simulink model "ar_lht_hw_target"  (R2018a)
settings: Solver=VariableStepAuto  StartTime=0.0  StopTime=ts*4+(526+25)*4*T  RelTol=1e-3  EnableMultiTasking=on
PreLoadFcn:
  | currentDir  = pwd;
  | filesepIdx   = strfind(currentDir, filesep);
  | newDir = currentDir(1:filesepIdx(end)-7);
  | 
  | addpath([newDir, '\scripts']);
InitFcn:
  | setup;
  | pre_processing;
values from neighbouring files (symbols this model uses):
  deltaTheta = 1    [setup.m]
  fps = f/((height)*(width))    (= 184.377034505)    [setup.m]
  height = 768    [setup.m]
  K = (maxTheta + deltaTheta)/R    (= 45)    [setup.m]
  maxRho = ceil(sqrt((height/2)^2+(width/2)^2))    [setup.m]
  maxTheta = 179    [setup.m]
  R = 4    [setup.m]
  T = 1/f    (= 6.89655172414e-09)    [setup.m]
  width = 1024    [setup.m]
libraries: xbsIndex_r4 x220, hdlsllib x6, visionhdlio x1, visionsources x1
(part 1 of 2)
settings Model: Creator=David Northcote  LastModifiedBy=rgb11127
settings OptimizationCC: LifeSpan=inf
settings DebuggingCC: SFUnexpectedBacktrackingDiag=warning  SFNoUnconditionalDefaultTransitionDiag=warning  SFExecutionAtInitializationDiag=none
settings CodeAppCC: StateflowObjectComments=on
settings GRTTargetCC: TargetLangStandard=C89/C90 (ANSI)  GeneratePreprocessorConditionals=Disable all
settings ConfigComp: CovMetricSettings=dw  CovHtmlReporting=on  CovSaveCumulativeToWorkspaceVar=on  CovSaveSingleToWorkspaceVar=on  CovExternalEMLEnable=off

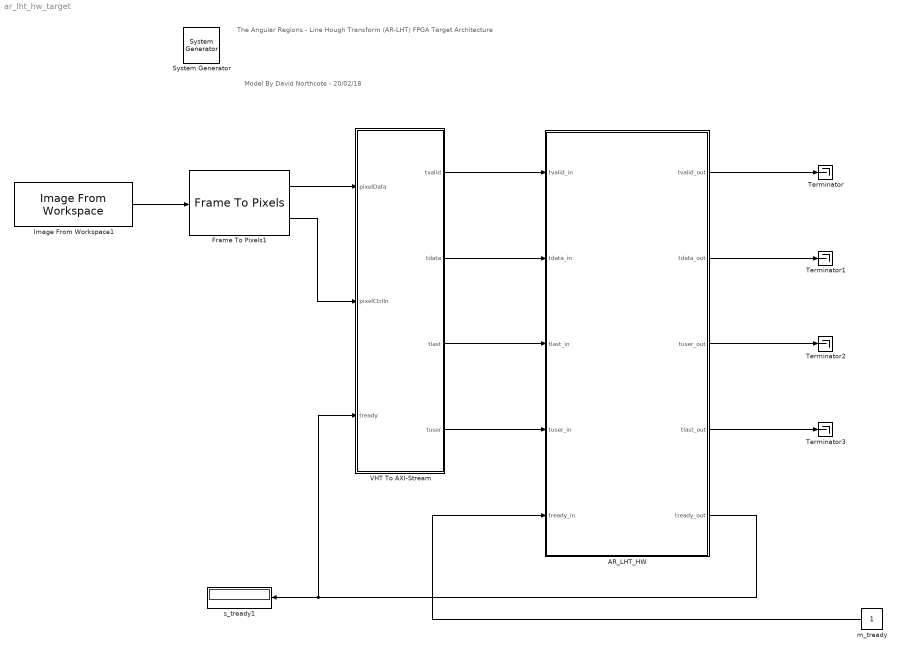
== system ar_lht_hw_target ==
  note: Model By David Northcote - 20/02/18
  note: The Angular Regions - Line Hough Transform (AR-LHT)
      | FPGA Target Architecture
  " System Generator" : xbsIndex_r4/ System Generator  Tag=genX  xilinxfamily=zynq  part=xc7z010  speed=-1  package=clg400  synthesis_tool=Vivado  clock_wrapper=Clock Enables  directory=./netlist  proj_type=Vivado  Synth_file=Vivado Synthesis Defaults  Impl_file=Vivado Implementation Defaults  testbench=off  simulink_period=T  sysclk_period=T*1e9  dcm_input_clock_period=10  incr_netlist=off  trim_vbits=Everywhere in SubSystem  dbl_ovrd=According to Block Masks  core_generation=According to Block Masks  run_coregen=off  deprecated_control=off  eval_field=0  block_type=sysgen
  AR_LHT_HW : Subsystem
  Frame To Pixels1 : visionhdlio/Frame To Pixels  NumComponents=1  VideoFormat=Custom  ActivePixelsPerLine=width  ActiveVideoLines=height  TotalPixelsPerLine=width  TotalVideoLines=height  StartingActiveLine=1  FrontPorch=0  SampleTime=0
      settings: SourceProductName=Vision HDL Toolbox  SourceProductBaseCode=VT
  Image From Workspace1 : visionsources/Image From Workspace  Tag=vipblks_nd  ImageValue=InputImage  Ts=1/fps  imagePorts=One multidimensional signal  OutPortLabels=R|G|B  ImageDataType=Inherit from 'Value'  Signed=on  WordLength=16  sdImageDataType=sfix(16)  FractionLengthMode=User-defined  FractionLength=15
      settings: SourceProductName=Computer Vision System Toolbox  SourceProductBaseCode=VP
  Terminator{,1..3} (4 alike) : Terminator
  VHT To AXI-Stream : Subsystem
  m_tready : Constant  OutDataTypeStr=boolean  SampleTime=T
  s_tready1 : Display
  wires:
  m_tready/1 -> AR_LHT_HW/5(tready_in)
  AR_LHT_HW/4(tlast_out) -> Terminator3/1
  AR_LHT_HW/3(tuser_out) -> Terminator2/1
  AR_LHT_HW/2(tdata_out) -> Terminator1/1
  AR_LHT_HW/1(tvalid_out) -> Terminator/1
  AR_LHT_HW/5(tready_out) -> s_tready1/1, VHT To AXI-Stream/3(tready)
  VHT To AXI-Stream/1(tvalid) -> AR_LHT_HW/1(tvalid_in)
  VHT To AXI-Stream/3(tlast) -> AR_LHT_HW/3(tlast_in)
  VHT To AXI-Stream/2(tdata) -> AR_LHT_HW/2(tdata_in)
  VHT To AXI-Stream/4(tuser) -> AR_LHT_HW/4(tuser_in)
  Frame To Pixels1/1 -> VHT To AXI-Stream/1(pixelData)
  Frame To Pixels1/2 -> VHT To AXI-Stream/2(pixelCtrlIn)
  Image From Workspace1/1 -> Frame To Pixels1/1

== system ar_lht_hw_target/AR_LHT_HW ==
  tvalid_in : Inport
  tdata_in : Inport  Port=2
  tlast_in : Inport  Port=3
  tuser_in : Inport  Port=4
  tready_in : Inport  Port=5
  DUT : Subsystem
  M_AXIS : Subsystem
  S_AXIS : Subsystem
  tvalid_out : Outport
  tdata_out : Outport  Port=2
  tuser_out : Outport  Port=3
  tlast_out : Outport  Port=4
  tready_out : Outport  Port=5
  wires:
  DUT/5(tready_out) -> S_AXIS/5(tready_in)
  M_AXIS/1(tready_out) -> DUT/5(tready_in)
  DUT/1(tvalid_out) -> M_AXIS/1(tvalid_in)
  DUT/2(tdata_out) -> M_AXIS/2(tdata_in)
  DUT/3(tlast_out) -> M_AXIS/3(tlast_in)
  DUT/4(tuser_out) -> M_AXIS/4(tuser_in)
  S_AXIS/2(tdata_out) -> DUT/2(tdata_in)
  S_AXIS/1(tvalid_out) -> DUT/1(tvalid_in)
  S_AXIS/3(tlast_out) -> DUT/3(tlast_in)
  S_AXIS/4(tuser_out) -> DUT/4(tuser_in)
  M_AXIS/4(tuser_out) -> tuser_out/1
  S_AXIS/5(tready_out) -> tready_out/1
  M_AXIS/5(tlast_out) -> tlast_out/1
  M_AXIS/3(tdata_out) -> tdata_out/1
  tready_in/1 -> M_AXIS/5(tready_in)
  M_AXIS/2(tvalid_out) -> tvalid_out/1
  tlast_in/1 -> S_AXIS/3(tlast_in)
  tvalid_in/1 -> S_AXIS/1(tvalid_in)
  tuser_in/1 -> S_AXIS/4(tuser_in)
  tdata_in/1 -> S_AXIS/2(tdata_in)

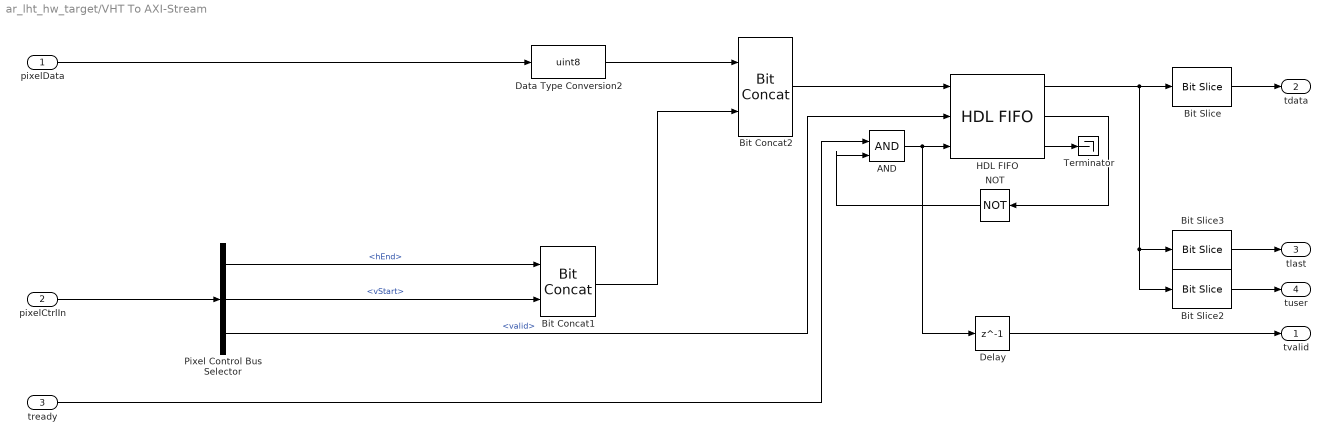
== system ar_lht_hw_target/VHT To AXI-Stream ==
  pixelData : Inport
  pixelCtrlIn : Inport  Port=2
  tready : Inport  Port=3
  AND : Logic  IconShape=distinctive  AllPortsSameDT=off  OutDataTypeStr=boolean
  Bit Concat1 : hdlsllib/Logic and Bit Operations/Bit Concat  numInputs=2
      settings: SourceProductName=HDL Coder  SourceProductBaseCode=HD
  Bit Concat2 : hdlsllib/Logic and Bit Operations/Bit Concat  numInputs=2
      settings: SourceProductName=HDL Coder  SourceProductBaseCode=HD
  Bit Slice : hdlsllib/Logic and Bit Operations/Bit Slice  lidx=9  ridx=2
  Bit Slice2 : hdlsllib/Logic and Bit Operations/Bit Slice  lidx=0  ridx=0
  Bit Slice3 : hdlsllib/Logic and Bit Operations/Bit Slice  lidx=1  ridx=1
  Data Type Conversion2 : DataTypeConversion  OutDataTypeStr=uint8
  Delay : Delay  DelayLength=1
  HDL FIFO : hdlsllib/HDL RAMs/HDL FIFO  fifo_size=1024  ratio=1  push_msg=Error  pop_msg=Error  show_empty=on  show_full=on  show_num=off
      settings: SourceProductName=HDL Coder  SourceProductBaseCode=HD
  NOT : Logic  Operator=NOT  IconShape=distinctive  AllPortsSameDT=off  OutDataTypeStr=boolean
  Pixel Control Bus Selector : BusSelector  OutputSignals=hEnd,vStart,valid
  Terminator : Terminator
  tvalid : Outport
  tdata : Outport  Port=2
  tlast : Outport  Port=3
  tuser : Outport  Port=4
  wires:
  pixelData/1 -> Data Type Conversion2/1
  pixelCtrlIn/1 -> Pixel Control Bus Selector/1
  Bit Concat2/1 -> HDL FIFO/1
  Data Type Conversion2/1 -> Bit Concat2/1
  Bit Concat1/1 -> Bit Concat2/2
  HDL FIFO/1 -> Bit Slice3/1, Bit Slice2/1, Bit Slice/1
  tready/1 -> AND/1
  HDL FIFO/2 -> NOT/1
  NOT/1 -> AND/2
  Bit Slice/1 -> tdata/1
  Bit Slice3/1 -> tlast/1
  Bit Slice2/1 -> tuser/1
  AND/1 -> Delay/1, HDL FIFO/3
  Pixel Control Bus Selector/1 -> Bit Concat1/1  "<hEnd>"
  Pixel Control Bus Selector/2 -> Bit Concat1/2  "<vStart>"
  Pixel Control Bus Selector/3 -> HDL FIFO/2  "<valid>"
  Delay/1 -> tvalid/1
  HDL FIFO/3 -> Terminator/1

== system ar_lht_hw_target/AR_LHT_HW/DUT ==
  tvalid_in : Inport
  tdata_in : Inport  Port=2
  tlast_in : Inport  Port=3
  tuser_in : Inport  Port=4
  tready_in : Inport  Port=5
  AXI FIFO : xbsIndex_r4/AXI FIFO  input_depth_axis=16  actual_fifo_depth_label=18  enable_tdata=on  enable_tdest=off  enable_tstrb=off  enable_tready=on  enable_tid=off  enable_tuser=on  enable_tkeep=off  enable_tlast=on  has_aresetn=off  enable_data_counts_axis=off  fifo_implementation_type_axis=Common Clock Distributed RAM  trim_axipin_name=on  programmable_full_type_axis=Full  full_threshold_assert_value_axis=0  programmable_empty_type_axis=Empty  empty_threshold_assert_value_axis=1022  underflow_flag_axi=0  underflow_sense_axi=Active High  overflow_flag_axi=0  overflow_sense_axi=Active High  block_type=axi_fifo
  Algorithm : Subsystem
  tvalid_out : Outport
  tdata_out : Outport  Port=2
  tlast_out : Outport  Port=3
  tuser_out : Outport  Port=4
  tready_out : Outport  Port=5
  wires:
  tvalid_in/1 -> Algorithm/2(tvalid_in)
  tready_in/1 -> Algorithm/1(tready_in)
  tlast_in/1 -> Algorithm/4(tlast_in)
  tuser_in/1 -> Algorithm/5(tuser_in)
  tdata_in/1 -> Algorithm/3(tdata_in)
  AXI FIFO/4 -> tuser_out/1
  AXI FIFO/3 -> tlast_out/1
  AXI FIFO/1 -> tvalid_out/1
  AXI FIFO/2 -> tdata_out/1
  AXI FIFO/5 -> tready_out/1
  Algorithm/5(tuser_out) -> AXI FIFO/5
  Algorithm/4(tlast_out) -> AXI FIFO/4
  Algorithm/3(tdata_out) -> AXI FIFO/3
  Algorithm/2(tvalid_out) -> AXI FIFO/2
  Algorithm/1(tready_out) -> AXI FIFO/1

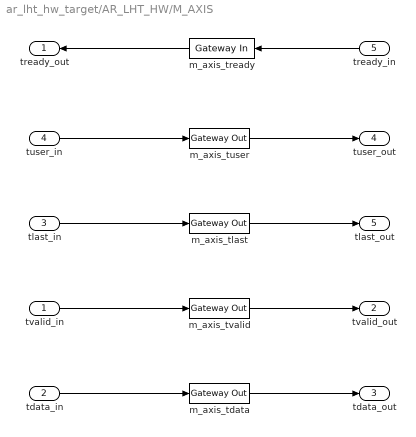
== system ar_lht_hw_target/AR_LHT_HW/M_AXIS ==
  tvalid_in : Inport
  tdata_in : Inport  Port=2
  tlast_in : Inport  Port=3
  tuser_in : Inport  Port=4
  tready_in : Inport  Port=5
  m_axis_tdata : xbsIndex_r4/Gateway Out  inherit_from_input=on  hdl_port=on  rows=1  columns=1  UseAsDAC=off  DACChannel='1'  interface=None  automatic_assignment=on  address_offset=hex2dec('00')  intf_name=''  intf_description=''  timing_constraint=None  locs_specified=off  LOCs={}  io_standard={}  block_type=gatewayout
  m_axis_tlast : xbsIndex_r4/Gateway Out  inherit_from_input=off  hdl_port=on  rows=1  columns=1  UseAsDAC=off  DACChannel='1'  interface=None  automatic_assignment=on  address_offset=hex2dec('00')  intf_name=''  intf_description=''  timing_constraint=None  locs_specified=off  LOCs={}  io_standard={}  block_type=gatewayout
  m_axis_tready : xbsIndex_r4/Gateway In  gui_display_data_type=Boolean  arith_type=Boolean  n_bits=16  bin_pt=14  preci_type=Single  exp_width=8  frac_width=24  rows=1  columns=1  quantization="Round  (unbiased: +/- Inf)"  overflow=Saturate  period=T  UseAsADC=off  ADCChannel='1'  interface=None  automatic_assignment=on  address_offset=hex2dec('00')  intf_name=''  intf_description=''  default_value=0  timing_constraint=None  locs_specified=off  LOCs={}  io_standard={}  inherit_from_input=off  hdl_port=on  dbl_ovrd=off  block_type=gatewayin
  m_axis_tuser : xbsIndex_r4/Gateway Out  inherit_from_input=off  hdl_port=on  rows=1  columns=1  UseAsDAC=off  DACChannel='1'  interface=None  automatic_assignment=on  address_offset=hex2dec('00')  intf_name=''  intf_description=''  timing_constraint=None  locs_specified=off  LOCs={}  io_standard={}  block_type=gatewayout
  m_axis_tvalid : xbsIndex_r4/Gateway Out  inherit_from_input=off  hdl_port=on  rows=1  columns=1  UseAsDAC=off  DACChannel='1'  interface=None  automatic_assignment=on  address_offset=hex2dec('00')  intf_name=''  intf_description=''  timing_constraint=None  locs_specified=off  LOCs={}  io_standard={}  block_type=gatewayout
  tready_out : Outport
  tvalid_out : Outport  Port=2
  tdata_out : Outport  Port=3
  tuser_out : Outport  Port=4
  tlast_out : Outport  Port=5
  wires:
  tuser_in/1 -> m_axis_tuser/1
  m_axis_tready/1 -> tready_out/1
  tlast_in/1 -> m_axis_tlast/1
  tdata_in/1 -> m_axis_tdata/1
  m_axis_tlast/1 -> tlast_out/1
  tvalid_in/1 -> m_axis_tvalid/1
  tready_in/1 -> m_axis_tready/1
  m_axis_tdata/1 -> tdata_out/1
  m_axis_tvalid/1 -> tvalid_out/1
  m_axis_tuser/1 -> tuser_out/1

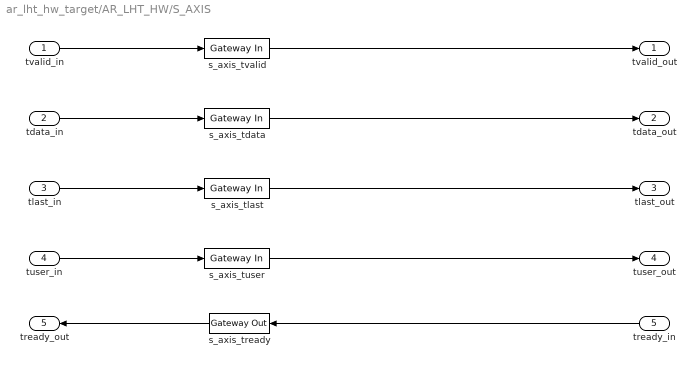
== system ar_lht_hw_target/AR_LHT_HW/S_AXIS ==
  tvalid_in : Inport
  tdata_in : Inport  Port=2
  tlast_in : Inport  Port=3
  tuser_in : Inport  Port=4
  tready_in : Inport  Port=5
  s_axis_tdata : xbsIndex_r4/Gateway In  gui_display_data_type=Fixed-point  arith_type=Unsigned  n_bits=8  bin_pt=0  preci_type=Single  exp_width=8  frac_width=24  rows=1  columns=1  quantization=Truncate  overflow=Flag as error  period=T  UseAsADC=off  ADCChannel='1'  interface=None  automatic_assignment=on  address_offset=hex2dec('00')  intf_name=''  intf_description=''  default_value=0  timing_constraint=None  locs_specified=off  LOCs={}  io_standard={}  inherit_from_input=off  hdl_port=on  dbl_ovrd=off  block_type=gatewayin
  s_axis_tlast : xbsIndex_r4/Gateway In  gui_display_data_type=Boolean  arith_type=Boolean  n_bits=32  bin_pt=0  preci_type=Single  exp_width=8  frac_width=24  rows=1  columns=1  quantization=Truncate  overflow=Flag as error  period=T  UseAsADC=off  ADCChannel='1'  interface=None  automatic_assignment=on  address_offset=hex2dec('00')  intf_name=''  intf_description=''  default_value=0  timing_constraint=None  locs_specified=off  LOCs={}  io_standard={}  inherit_from_input=off  hdl_port=on  dbl_ovrd=off  block_type=gatewayin
  s_axis_tready : xbsIndex_r4/Gateway Out  inherit_from_input=on  hdl_port=on  rows=1  columns=1  UseAsDAC=off  DACChannel='1'  interface=None  automatic_assignment=on  address_offset=hex2dec('00')  intf_name=''  intf_description=''  timing_constraint=None  locs_specified=off  LOCs={}  io_standard={}  block_type=gatewayout
  s_axis_tuser : xbsIndex_r4/Gateway In  gui_display_data_type=Boolean  arith_type=Boolean  n_bits=1  bin_pt=0  preci_type=Single  exp_width=8  frac_width=24  rows=1  columns=1  quantization=Truncate  overflow=Flag as error  period=T  UseAsADC=off  ADCChannel='1'  interface=None  automatic_assignment=on  address_offset=hex2dec('00')  intf_name=''  intf_description=''  default_value=0  timing_constraint=None  locs_specified=off  LOCs={}  io_standard={}  inherit_from_input=off  hdl_port=on  dbl_ovrd=off  block_type=gatewayin
  s_axis_tvalid : xbsIndex_r4/Gateway In  gui_display_data_type=Boolean  arith_type=Boolean  n_bits=32  bin_pt=0  preci_type=Single  exp_width=8  frac_width=24  rows=1  columns=1  quantization=Truncate  overflow=Flag as error  period=T  UseAsADC=off  ADCChannel='1'  interface=None  automatic_assignment=on  address_offset=hex2dec('00')  intf_name=''  intf_description=''  default_value=0  timing_constraint=None  locs_specified=off  LOCs={}  io_standard={}  inherit_from_input=off  hdl_port=on  dbl_ovrd=off  block_type=gatewayin
  tvalid_out : Outport
  tdata_out : Outport  Port=2
  tlast_out : Outport  Port=3
  tuser_out : Outport  Port=4
  tready_out : Outport  Port=5
  wires:
  s_axis_tuser/1 -> tuser_out/1
  s_axis_tlast/1 -> tlast_out/1
  s_axis_tdata/1 -> tdata_out/1
  s_axis_tvalid/1 -> tvalid_out/1
  tdata_in/1 -> s_axis_tdata/1
  tvalid_in/1 -> s_axis_tvalid/1
  tlast_in/1 -> s_axis_tlast/1
  tuser_in/1 -> s_axis_tuser/1
  tready_in/1 -> s_axis_tready/1
  s_axis_tready/1 -> tready_out/1

== system ar_lht_hw_target/AR_LHT_HW/DUT/Algorithm ==
  note: tready should never have any latency. It will only be used to pop the IP core's front-end FIFO.
  tready_in : Inport
  tvalid_in : Inport  Port=2
  tdata_in : Inport  Port=3
  tlast_in : Inport  Port=4
  tuser_in : Inport  Port=5
  AlgorithmDUT : Subsystem
  tready_out : Outport
  tvalid_out : Outport  Port=2
  tdata_out : Outport  Port=3
  tlast_out : Outport  Port=4
  tuser_out : Outport  Port=5
  wires:
  AlgorithmDUT/4(tvalid_out) -> tvalid_out/1
  AlgorithmDUT/3(tdata_out) -> tdata_out/1
  AlgorithmDUT/2(tlast_out) -> tlast_out/1
  AlgorithmDUT/1(tuser_out) -> tuser_out/1
  tdata_in/1 -> AlgorithmDUT/3(tdata_in)
  tlast_in/1 -> AlgorithmDUT/2(tlast_in)
  tuser_in/1 -> AlgorithmDUT/1(tuser_in)
  tvalid_in/1 -> AlgorithmDUT/4(tvalid_in)
  tready_in/1 -> tready_out/1

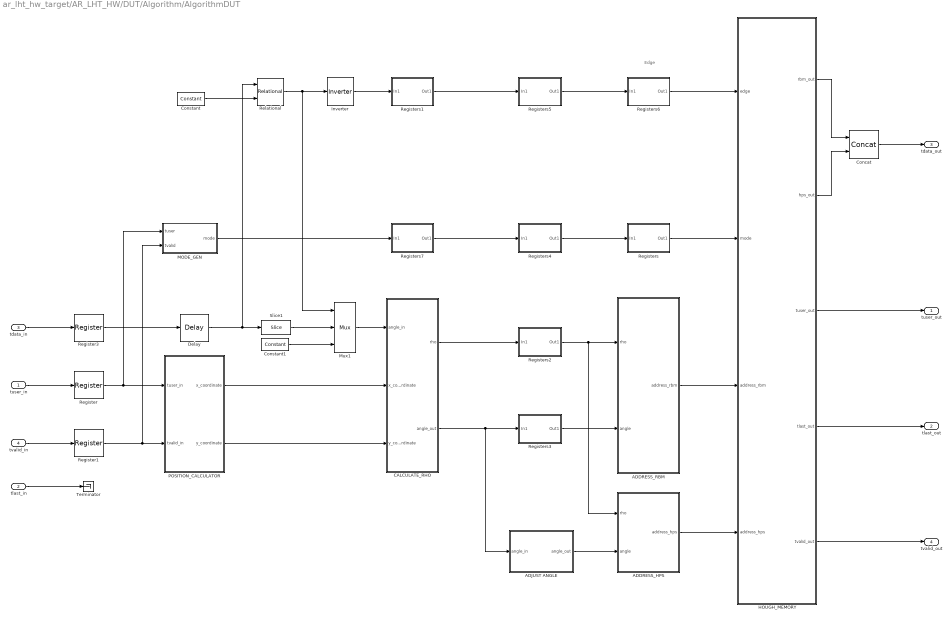
== system ar_lht_hw_target/AR_LHT_HW/DUT/Algorithm/AlgorithmDUT ==
  note: Edge
  tuser_in : Inport
  tlast_in : Inport  Port=2
  tdata_in : Inport  Port=3
  tvalid_in : Inport  Port=4
  ADDRESS_HPS : Subsystem
  ADDRESS_RBM : Subsystem
  ADJUST ANGLE : Subsystem
  CALCULATE_RHO : Subsystem
  Concat : xbsIndex_r4/Concat  num_inputs=2  dbl_ovrd=off  block_type=concat
  Constant : xbsIndex_r4/Constant  const=255  gui_display_data_type=Fixed-point  arith_type=Unsigned  n_bits=8  bin_pt=0  preci_type=Single  exp_width=8  frac_width=24  explicit_period=on  period=T  equ=P=C  opselect=C  inp2=PCIN>>17  opr=+  inp1=P  carry=CIN  dbl_ovrd=off  block_type=constant
  Constant1 : xbsIndex_r4/Constant  const=0  gui_display_data_type=Fixed-point  arith_type=Unsigned  n_bits=8  bin_pt=0  preci_type=Single  exp_width=8  frac_width=24  explicit_period=on  period=T  equ=P=C  opselect=C  inp2=PCIN>>17  opr=+  inp1=P  carry=CIN  dbl_ovrd=off  block_type=constant
  Delay : xbsIndex_r4/Delay  rst=off  infoeditControl=Selection of Reset will increase slice count due to use of real FFs and instead of SRLs  en=off  latency=1  reg_retiming=off  dbl_ovrd=off  block_type=delay
  HOUGH_MEMORY : Subsystem
  Inverter : xbsIndex_r4/Inverter  en=off  latency=0  dbl_ovrd=off  block_type=inv
  MODE_GEN : Subsystem
  Mux1 : xbsIndex_r4/Mux  inputs=2  en=off  latency=0  precision=Full  arith_type=Unsigned  n_bits=16  bin_pt=14  quantization=Truncate  overflow=Wrap  dbl_ovrd=off  block_type=mux
  POSITION_CALCULATOR : Subsystem
  Register : xbsIndex_r4/Register  init=0  rst=off  en=off  dbl_ovrd=off  block_type=register
  Register1 : xbsIndex_r4/Register  init=0  rst=off  en=off  dbl_ovrd=off  block_type=register
  Register3 : xbsIndex_r4/Register  init=0  rst=off  en=off  dbl_ovrd=off  block_type=register
  Registers : Subsystem
  Registers1 : Subsystem
  Registers2 : Subsystem
  Registers3 : Subsystem
  Registers4 : Subsystem
  Registers5 : Subsystem
  Registers6 : Subsystem
  Registers7 : Subsystem
  Relational : xbsIndex_r4/Relational  mode=a=b  op_type=Bool  en=off  latency=0  dbl_ovrd=off  block_type=relational
  Slice1 : xbsIndex_r4/Slice  nbits=8  boolean_output=off  mode=Two Bit Locations  bit1=7  base1=LSB of Input  bit0=0  base0=LSB of Input  dbl_ovrd=off  block_type=slice
  Terminator : Terminator
  tuser_out : Outport
  tlast_out : Outport  Port=2
  tdata_out : Outport  Port=3
  tvalid_out : Outport  Port=4
  wires:
  Concat/1 -> tdata_out/1
  HOUGH_MEMORY/3(tuser_out) -> tuser_out/1
  HOUGH_MEMORY/4(tlast_out) -> tlast_out/1
  tdata_in/1 -> Register3/1
  tuser_in/1 -> Register/1
  tvalid_in/1 -> Register1/1
  HOUGH_MEMORY/5(tvalid_out) -> tvalid_out/1
  HOUGH_MEMORY/1(rbm_out) -> Concat/1
  HOUGH_MEMORY/2(hps_out) -> Concat/2
  ADDRESS_HPS/1(address_hps) -> HOUGH_MEMORY/4(address_hps)
  ADDRESS_RBM/1(address_rbm) -> HOUGH_MEMORY/3(address_rbm)
  Registers/1(Out1) -> HOUGH_MEMORY/2(mode)
  Registers6/1(Out1) -> HOUGH_MEMORY/1(edge)
  Register1/1 -> POSITION_CALCULATOR/2(tvalid_in), MODE_GEN/2(tvalid)
  Registers4/1(Out1) -> Registers/1(In1)
  Registers7/1(Out1) -> Registers4/1(In1)
  MODE_GEN/1(mode) -> Registers7/1(In1)
  Inverter/1 -> Registers1/1(In1)
  Constant1/1 -> Mux1/3
  Slice1/1 -> Mux1/2
  Mux1/1 -> CALCULATE_RHO/1(angle_in)
  Constant/1 -> Relational/2
  tlast_in/1 -> Terminator/1
  POSITION_CALCULATOR/2(y_coordinate) -> CALCULATE_RHO/3(y_coordinate)
  POSITION_CALCULATOR/1(x_coordinate) -> CALCULATE_RHO/2(x_coordinate)
  CALCULATE_RHO/2(angle_out) -> ADJUST ANGLE/1(angle_in), Registers3/1(In1)
  ADJUST ANGLE/1(angle_out) -> ADDRESS_HPS/2(angle)
  Registers3/1(Out1) -> ADDRESS_RBM/2(angle)
  Registers2/1(Out1) -> ADDRESS_HPS/1(rho), ADDRESS_RBM/1(rho)
  CALCULATE_RHO/1(rho) -> Registers2/1(In1)
  Register/1 -> POSITION_CALCULATOR/1(tuser_in), MODE_GEN/1(tuser)
  Register3/1 -> Delay/1
  Relational/1 -> Inverter/1, Mux1/1
  Registers5/1(Out1) -> Registers6/1(In1)
  Registers1/1(Out1) -> Registers5/1(In1)
  Delay/1 -> Slice1/1, Relational/1

== system ar_lht_hw_target/AR_LHT_HW/DUT/Algorithm/AlgorithmDUT/ADDRESS_HPS ==
  rho : Inport
  angle : Inport  Port=2
  AddSub1 : xbsIndex_r4/AddSub  mode=Addition  use_carryin=off  use_carryout=off  en=off  latency=1  precision=User Defined  arith_type=Unsigned  n_bits=ceil(log2(maxRho*2))  bin_pt=0  quantization=Truncate  overflow=Wrap  use_behavioral_HDL=on  hw_selection=Fabric  pipelined=on  dbl_ovrd=off  block_type=addsub
  AddSub2 : xbsIndex_r4/AddSub  mode=Addition  use_carryin=off  use_carryout=off  en=off  latency=1  precision=User Defined  arith_type=Unsigned  n_bits=ceil(log2(maxRho*2)+log2(K-1))  bin_pt=0  quantization=Truncate  overflow=Wrap  use_behavioral_HDL=on  hw_selection=Fabric  pipelined=on  dbl_ovrd=off  block_type=addsub
  CMult : xbsIndex_r4/CMult  const=maxRho*2  gui_display_data_type=Fixed-point  const_n_bits=ceil(log2(maxRho)+1)  const_bin_pt=0  float_type=Single  exp_bits=8  fraction_bits=24  en=off  latency=1  precision=Full  arith_type="Signed  (2's comp)"  n_bits=16  bin_pt=14  quantization=Truncate  overflow=Wrap  use_behavioral_HDL=off  mem_type=Distributed RAM  pipeline=off  dbl_ovrd=off  block_type=cmult
  rho_offset_general : xbsIndex_r4/Constant  const=maxRho-1  gui_display_data_type=Fixed-point  arith_type=Unsigned  n_bits=ceil(log2(maxRho-1))  bin_pt=0  preci_type=Single  exp_width=8  frac_width=24  explicit_period=on  period=T  equ=P=C  opselect=C  inp2=PCIN>>17  opr=+  inp1=P  carry=CIN  dbl_ovrd=off  block_type=constant
  address_hps : Outport
  wires:
  rho/1 -> AddSub1/2
  AddSub1/1 -> AddSub2/1
  rho_offset_general/1 -> AddSub1/1
  angle/1 -> CMult/1
  AddSub2/1 -> address_hps/1
  CMult/1 -> AddSub2/2

== system ar_lht_hw_target/AR_LHT_HW/DUT/Algorithm/AlgorithmDUT/ADDRESS_RBM ==
  rho : Inport
  angle : Inport  Port=2
  AddSub1 : xbsIndex_r4/AddSub  mode=Addition  use_carryin=off  use_carryout=off  en=off  latency=1  precision=User Defined  arith_type=Unsigned  n_bits=ceil(log2(maxRho*2))  bin_pt=0  quantization=Truncate  overflow=Saturate  use_behavioral_HDL=on  hw_selection=Fabric  pipelined=on  dbl_ovrd=off  block_type=addsub
  AddSub2 : xbsIndex_r4/AddSub  mode=Addition  use_carryin=off  use_carryout=off  en=off  latency=1  precision=User Defined  arith_type=Unsigned  n_bits=ceil(log2(maxRho*2)+log2(maxTheta))  bin_pt=0  quantization=Truncate  overflow=Wrap  use_behavioral_HDL=on  hw_selection=Fabric  pipelined=on  dbl_ovrd=off  block_type=addsub
  CMult : xbsIndex_r4/CMult  const=maxRho*2  gui_display_data_type=Fixed-point  const_n_bits=ceil(log2(maxRho)+1)  const_bin_pt=0  float_type=Single  exp_bits=8  fraction_bits=24  en=off  latency=1  precision=Full  arith_type="Signed  (2's comp)"  n_bits=16  bin_pt=14  quantization=Truncate  overflow=Wrap  use_behavioral_HDL=off  mem_type=Distributed RAM  pipeline=off  dbl_ovrd=off  block_type=cmult
  rho_offset_general : xbsIndex_r4/Constant  const=maxRho-1  gui_display_data_type=Fixed-point  arith_type=Unsigned  n_bits=ceil(log2(maxRho-1))  bin_pt=0  preci_type=Single  exp_width=8  frac_width=24  explicit_period=on  period=T  equ=P=C  opselect=C  inp2=PCIN>>17  opr=+  inp1=P  carry=CIN  dbl_ovrd=off  block_type=constant
  address_rbm : Outport
  wires:
  CMult/1 -> AddSub2/2
  AddSub2/1 -> address_rbm/1
  angle/1 -> CMult/1
  rho_offset_general/1 -> AddSub1/1
  AddSub1/1 -> AddSub2/1
  rho/1 -> AddSub1/2

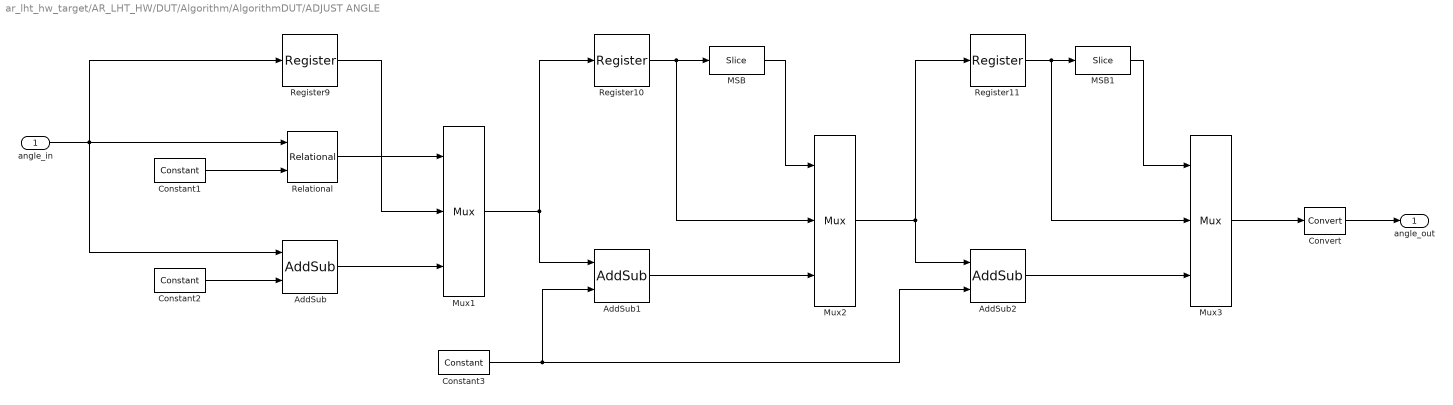
== system ar_lht_hw_target/AR_LHT_HW/DUT/Algorithm/AlgorithmDUT/ADJUST ANGLE ==
  angle_in : Inport
  AddSub : xbsIndex_r4/AddSub  mode=Subtraction  use_carryin=off  use_carryout=off  en=off  latency=1  precision=Full  arith_type=Unsigned  n_bits=16  bin_pt=14  quantization=Truncate  overflow=Wrap  use_behavioral_HDL=off  hw_selection=Fabric  pipelined=off  dbl_ovrd=off  block_type=addsub
  AddSub1 : xbsIndex_r4/AddSub  mode=Addition  use_carryin=off  use_carryout=off  en=off  latency=1  precision=Full  arith_type=Unsigned  n_bits=16  bin_pt=14  quantization=Truncate  overflow=Wrap  use_behavioral_HDL=off  hw_selection=Fabric  pipelined=off  dbl_ovrd=off  block_type=addsub
  AddSub2 : xbsIndex_r4/AddSub  mode=Addition  use_carryin=off  use_carryout=off  en=off  latency=1  precision=Full  arith_type=Unsigned  n_bits=16  bin_pt=14  quantization=Truncate  overflow=Wrap  use_behavioral_HDL=off  hw_selection=Fabric  pipelined=off  dbl_ovrd=off  block_type=addsub
  Constant1 : xbsIndex_r4/Constant  const=K-deltaTheta  gui_display_data_type=Fixed-point  arith_type=Unsigned  n_bits=ceil(log2(K-deltaTheta))  bin_pt=0  preci_type=Single  exp_width=8  frac_width=24  explicit_period=on  period=T  equ=P=C  opselect=C  inp2=PCIN>>17  opr=+  inp1=P  carry=CIN  dbl_ovrd=off  block_type=constant
  Constant2 : xbsIndex_r4/Constant  const=maxTheta + deltaTheta - K  gui_display_data_type=Fixed-point  arith_type=Unsigned  n_bits=ceil(log2(maxTheta - K))  bin_pt=0  preci_type=Single  exp_width=8  frac_width=24  explicit_period=on  period=T  equ=P=C  opselect=C  inp2=PCIN>>17  opr=+  inp1=P  carry=CIN  dbl_ovrd=off  block_type=constant
  Constant3 : xbsIndex_r4/Constant  const=K  gui_display_data_type=Fixed-point  arith_type=Unsigned  n_bits=ceil(log2(K))  bin_pt=0  preci_type=Single  exp_width=8  frac_width=24  explicit_period=on  period=T  equ=P=C  opselect=C  inp2=PCIN>>17  opr=+  inp1=P  carry=CIN  dbl_ovrd=off  block_type=constant
  Convert : xbsIndex_r4/Convert  gui_display_data_type=Fixed-point  arith_type=Unsigned  n_bits=ceil(log2(K-deltaTheta))  bin_pt=0  float_type=Single  exp_bits=8  fraction_bits=24  quantization=Truncate  overflow=Wrap  en=off  latency=0  pipeline=off  dbl_ovrd=off  block_type=convert
  MSB : xbsIndex_r4/Slice  nbits=8  boolean_output=on  mode=Upper Bit Location + Width  bit1=0  base1=MSB of Input  bit0=24  base0=LSB of Input  dbl_ovrd=off  block_type=slice
  MSB1 : xbsIndex_r4/Slice  nbits=8  boolean_output=on  mode=Upper Bit Location + Width  bit1=0  base1=MSB of Input  bit0=24  base0=LSB of Input  dbl_ovrd=off  block_type=slice
  Mux1 : xbsIndex_r4/Mux  inputs=2  en=off  latency=0  precision=Full  arith_type=Unsigned  n_bits=16  bin_pt=14  quantization=Truncate  overflow=Wrap  dbl_ovrd=off  block_type=mux
  Mux2 : xbsIndex_r4/Mux  inputs=2  en=off  latency=0  precision=Full  arith_type=Unsigned  n_bits=16  bin_pt=14  quantization=Truncate  overflow=Wrap  dbl_ovrd=off  block_type=mux
  Mux3 : xbsIndex_r4/Mux  inputs=2  en=off  latency=0  precision=Full  arith_type=Unsigned  n_bits=16  bin_pt=14  quantization=Truncate  overflow=Wrap  dbl_ovrd=off  block_type=mux
  Register10 : xbsIndex_r4/Register  init=0  rst=off  en=off  dbl_ovrd=off  block_type=register
  Register11 : xbsIndex_r4/Register  init=0  rst=off  en=off  dbl_ovrd=off  block_type=register
  Register9 : xbsIndex_r4/Register  init=0  rst=off  en=off  dbl_ovrd=off  block_type=register
  Relational : xbsIndex_r4/Relational  mode=a>b  op_type=Bool  en=off  latency=1  dbl_ovrd=off  block_type=relational
  angle_out : Outport
  wires:
  angle_in/1 -> AddSub/1, Relational/1, Register9/1
  AddSub1/1 -> Mux2/3
  Relational/1 -> Mux1/1
  Register10/1 -> Mux2/2, MSB/1
  Mux1/1 -> Register10/1, AddSub1/1
  Constant1/1 -> Relational/2
  MSB/1 -> Mux2/1
  Mux3/1 -> Convert/1
  AddSub/1 -> Mux1/3
  Register11/1 -> MSB1/1, Mux3/2
  MSB1/1 -> Mux3/1
  AddSub2/1 -> Mux3/3
  Mux2/1 -> Register11/1, AddSub2/1
  Constant3/1 -> AddSub2/2, AddSub1/2
  Constant2/1 -> AddSub/2
  Register9/1 -> Mux1/2
  Convert/1 -> angle_out/1

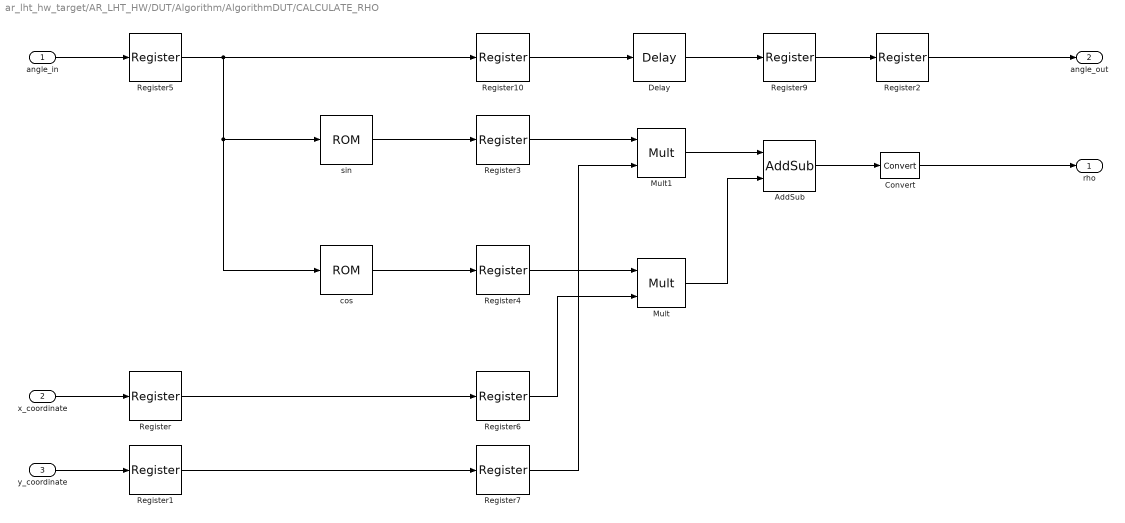
== system ar_lht_hw_target/AR_LHT_HW/DUT/Algorithm/AlgorithmDUT/CALCULATE_RHO ==
  angle_in : Inport
  x_coordinate : Inport  Port=2
  y_coordinate : Inport  Port=3
  AddSub : xbsIndex_r4/AddSub  mode=Addition  use_carryin=off  use_carryout=off  en=off  latency=1  precision=Full  arith_type="Signed  (2's comp)"  n_bits=ceil(log2(maxRho)+1)  bin_pt=0  quantization="Round  (unbiased: +/- Inf)"  overflow=Saturate  use_behavioral_HDL=on  hw_selection=Fabric  pipelined=on  dbl_ovrd=off  block_type=addsub
  Convert : xbsIndex_r4/Convert  gui_display_data_type=Fixed-point  arith_type="Signed  (2's comp)"  n_bits=ceil(log2(maxRho)+1)  bin_pt=0  float_type=Single  exp_bits=8  fraction_bits=24  quantization="Round  (unbiased: +/- Inf)"  overflow=Saturate  en=off  latency=1  pipeline=off  dbl_ovrd=off  block_type=convert
  Delay : xbsIndex_r4/Delay  rst=off  infoeditControl=Selection of Reset will increase slice count due to use of real FFs and instead of SRLs  en=off  latency=3  reg_retiming=off  dbl_ovrd=off  block_type=delay
  Mult : xbsIndex_r4/Mult  precision=Full  arith_type="Signed  (2's comp)"  n_bits=16  bin_pt=14  quantization=Truncate  overflow=Wrap  en=off  latency=3  use_behavioral_HDL=off  opt=Area  use_embedded=off  optimum_pipeline=off  pipeline=on  dbl_ovrd=off  use_rpm=on  placement_style=Triangular  block_type=mult
  Mult1 : xbsIndex_r4/Mult  precision=Full  arith_type="Signed  (2's comp)"  n_bits=16  bin_pt=14  quantization=Truncate  overflow=Wrap  en=off  latency=3  use_behavioral_HDL=off  opt=Area  use_embedded=off  optimum_pipeline=off  pipeline=on  dbl_ovrd=off  use_rpm=on  placement_style=Triangular  block_type=mult
  Register{,1..7,9..10} (10 alike) : xbsIndex_r4/Register  init=0  rst=off  en=off  dbl_ovrd=off  block_type=register
  cos : xbsIndex_r4/ROM  depth=maxTheta+deltaTheta  initVector=cos(deg2rad([0:1:maxTheta]))  distributed_mem=Distributed memory  rst=off  init_reg=0  en=off  latency=0  gui_display_data_type=Fixed-point  arith_type="Signed  (2's comp)"  n_bits=14  bin_pt=13  preci_type=Single  exp_width=8  frac_width=24  optimize=Area  use_rpm=on  dbl_ovrd=off  block_type=sprom
  sin : xbsIndex_r4/ROM  depth=maxTheta+deltaTheta  initVector=sin(deg2rad([0:1:maxTheta]))  distributed_mem=Distributed memory  rst=off  init_reg=0  en=off  latency=0  gui_display_data_type=Fixed-point  arith_type="Signed  (2's comp)"  n_bits=14  bin_pt=13  preci_type=Single  exp_width=8  frac_width=24  optimize=Area  use_rpm=off  dbl_ovrd=off  block_type=sprom
  rho : Outport
  angle_out : Outport  Port=2
  wires:
  AddSub/1 -> Convert/1
  Register4/1 -> Mult/1
  Register3/1 -> Mult1/1
  Register5/1 -> Register10/1, cos/1, sin/1
  Register1/1 -> Register7/1
  Register/1 -> Register6/1
  angle_in/1 -> Register5/1
  sin/1 -> Register3/1
  y_coordinate/1 -> Register1/1
  Mult/1 -> AddSub/2
  cos/1 -> Register4/1
  Mult1/1 -> AddSub/1
  x_coordinate/1 -> Register/1
  Register9/1 -> Register2/1
  Register10/1 -> Delay/1
  Delay/1 -> Register9/1
  Register6/1 -> Mult/2
  Register7/1 -> Mult1/2
  Register2/1 -> angle_out/1
  Convert/1 -> rho/1

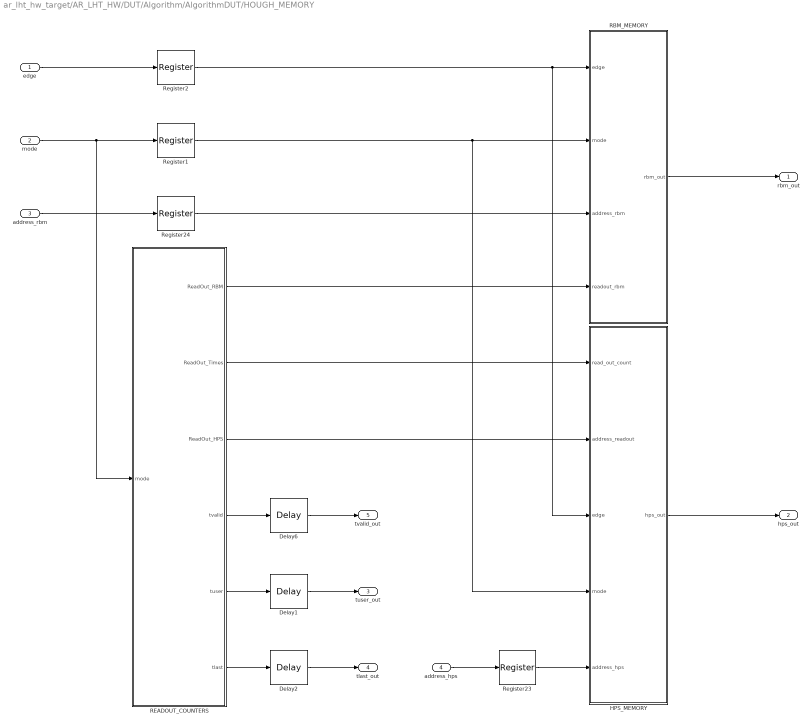
== system ar_lht_hw_target/AR_LHT_HW/DUT/Algorithm/AlgorithmDUT/HOUGH_MEMORY ==
  edge : Inport
  mode : Inport  Port=2
  address_rbm : Inport  Port=3
  address_hps : Inport  Port=4
  Delay1 : xbsIndex_r4/Delay  rst=off  infoeditControl=Selection of Reset will increase slice count due to use of real FFs and instead of SRLs  en=off  latency=13  reg_retiming=off  dbl_ovrd=off  block_type=delay
  Delay2 : xbsIndex_r4/Delay  rst=off  infoeditControl=Selection of Reset will increase slice count due to use of real FFs and instead of SRLs  en=off  latency=13  reg_retiming=off  dbl_ovrd=off  block_type=delay
  Delay6 : xbsIndex_r4/Delay  rst=off  infoeditControl=Selection of Reset will increase slice count due to use of real FFs and instead of SRLs  en=off  latency=13  reg_retiming=off  dbl_ovrd=off  block_type=delay
  HPS_MEMORY : Subsystem
  RBM_MEMORY : Subsystem
  READOUT_COUNTERS : Subsystem
  Register{1..2,23..24} (4 alike) : xbsIndex_r4/Register  init=0  rst=off  en=off  dbl_ovrd=off  block_type=register
  rbm_out : Outport
  hps_out : Outport  Port=2
  tuser_out : Outport  Port=3
  tlast_out : Outport  Port=4
  tvalid_out : Outport  Port=5
  wires:
  READOUT_COUNTERS/6(tlast) -> Delay2/1
  Register1/1 -> RBM_MEMORY/2(mode), HPS_MEMORY/4(mode)
  Register24/1 -> RBM_MEMORY/3(address_rbm)
  READOUT_COUNTERS/5(tuser) -> Delay1/1
  Register2/1 -> HPS_MEMORY/3(edge), RBM_MEMORY/1(edge)
  Delay6/1 -> tvalid_out/1
  address_hps/1 -> Register23/1
  READOUT_COUNTERS/1(ReadOut_RBM) -> RBM_MEMORY/4(readout_rbm)
  READOUT_COUNTERS/2(ReadOut_Times) -> HPS_MEMORY/1(read_out_count)
  address_rbm/1 -> Register24/1
  mode/1 -> Register1/1, READOUT_COUNTERS/1(mode)
  READOUT_COUNTERS/3(ReadOut_HPS) -> HPS_MEMORY/2(address_readout)
  edge/1 -> Register2/1
  READOUT_COUNTERS/4(tvalid) -> Delay6/1
  Register23/1 -> HPS_MEMORY/5(address_hps)
  Delay2/1 -> tlast_out/1
  HPS_MEMORY/1(hps_out) -> hps_out/1
  RBM_MEMORY/1(rbm_out) -> rbm_out/1
  Delay1/1 -> tuser_out/1

== system ar_lht_hw_target/AR_LHT_HW/DUT/Algorithm/AlgorithmDUT/MODE_GEN ==
  tuser : Inport
  tvalid : Inport  Port=2
  Assert : xbsIndex_r4/Assert  assert_type=on  type_source=Explicitly  gui_display_data_type=Boolean  arith_type=Boolean  n_bits=16  bin_pt=14  preci_type=Single  exp_width=8  frac_width=24  assert_rate=on  rate_source=Explicitly  period=T  output_port=on  block_type=assert
  Logical : xbsIndex_r4/Logical  logical_function=NOR  inputs=2  en=off  latency=0  precision=Full  arith_type=Unsigned  n_bits=16  bin_pt=0  align_bp=on  dbl_ovrd=off  block_type=logical
  Logical1 : xbsIndex_r4/Logical  logical_function=AND  inputs=2  en=off  latency=0  precision=Full  arith_type=Unsigned  n_bits=16  bin_pt=0  align_bp=on  dbl_ovrd=off  block_type=logical
  Register13 : xbsIndex_r4/Register  init=0  rst=off  en=on  dbl_ovrd=off  block_type=register
  Register14 : xbsIndex_r4/Register  init=0  rst=off  en=on  dbl_ovrd=off  block_type=register
  mode : Outport
  wires:
  Register14/1 -> Logical/1, Logical/2
  Logical/1 -> Register13/1
  Logical1/1 -> Register13/2
  Register13/1 -> Assert/1
  tvalid/1 -> Register14/2, Logical1/2
  tuser/1 -> Logical1/1
  Assert/1 -> mode/1, Register14/1

== system ar_lht_hw_target/AR_LHT_HW/DUT/Algorithm/AlgorithmDUT/POSITION_CALCULATOR ==
  tuser_in : Inport
  tvalid_in : Inport  Port=2
  Constant1 : xbsIndex_r4/Constant  const=width/2-2  gui_display_data_type=Fixed-point  arith_type=Unsigned  n_bits=ceil(log2(width/2-2))  bin_pt=0  preci_type=Single  exp_width=8  frac_width=24  explicit_period=on  period=T  equ=P=C  opselect=C  inp2=PCIN>>17  opr=+  inp1=P  carry=CIN  dbl_ovrd=off  block_type=constant
  Logical : xbsIndex_r4/Logical  logical_function=AND  inputs=2  en=off  latency=0  precision=Full  arith_type=Unsigned  n_bits=16  bin_pt=0  align_bp=on  dbl_ovrd=off  block_type=logical
  Relational : xbsIndex_r4/Relational  mode=a=b  op_type=Bool  en=on  latency=1  dbl_ovrd=off  block_type=relational
  x_counter : xbsIndex_r4/Counter  cnt_type=Count Limited  cnt_to=width/2-1  operation=Up  start_count=-width/2  cnt_by_val=1  arith_type="Signed  (2's comp)"  n_bits=ceil(log2(width/2-1)+1)  bin_pt=0  load_pin=off  rst=on  en=on  explicit_period=on  period=T  use_behavioral_HDL=on  implementation=Fabric  dbl_ovrd=off  block_type=counter
  y_counter : xbsIndex_r4/Counter  cnt_type=Count Limited  cnt_to=height/2-1  operation=Up  start_count=-height/2  cnt_by_val=1  arith_type="Signed  (2's comp)"  n_bits=ceil(log2(height/2-1)+1)  bin_pt=0  load_pin=off  rst=on  en=on  explicit_period=on  period=T  use_behavioral_HDL=on  implementation=Fabric  dbl_ovrd=off  block_type=counter
  x_coordinate : Outport
  y_coordinate : Outport  Port=2
  wires:
  Constant1/1 -> Relational/2
  tuser_in/1 -> y_counter/1, x_counter/1
  y_counter/1 -> y_coordinate/1
  x_counter/1 -> Relational/1, x_coordinate/1
  Logical/1 -> y_counter/2
  Relational/1 -> Logical/1
  tvalid_in/1 -> Logical/2, x_counter/2, Relational/3

== system ar_lht_hw_target/AR_LHT_HW/DUT/Algorithm/AlgorithmDUT/Registers ==
  In1 : Inport
  Register5 : xbsIndex_r4/Register  init=0  rst=off  en=off  dbl_ovrd=off  block_type=register
  Register7 : xbsIndex_r4/Register  init=0  rst=off  en=off  dbl_ovrd=off  block_type=register
  Out1 : Outport
  wires:
  Register5/1 -> Register7/1
  In1/1 -> Register5/1
  Register7/1 -> Out1/1

== system ar_lht_hw_target/AR_LHT_HW/DUT/Algorithm/AlgorithmDUT/Registers1 ==
  In1 : Inport
  Register{1..7} (7 alike) : xbsIndex_r4/Register  init=0  rst=off  en=off  dbl_ovrd=off  block_type=register
  Out1 : Outport
  wires:
  Register1/1 -> Register5/1
  Register5/1 -> Register7/1
  In1/1 -> Register4/1
  Register7/1 -> Register6/1
  Register2/1 -> Register1/1
  Register3/1 -> Register2/1
  Register4/1 -> Register3/1
  Register6/1 -> Out1/1

== system ar_lht_hw_target/AR_LHT_HW/DUT/Algorithm/AlgorithmDUT/Registers2 ==
  In1 : Inport
  Register1 : xbsIndex_r4/Register  init=0  rst=off  en=off  dbl_ovrd=off  block_type=register
  Register5 : xbsIndex_r4/Register  init=0  rst=off  en=off  dbl_ovrd=off  block_type=register
  Register7 : xbsIndex_r4/Register  init=0  rst=off  en=off  dbl_ovrd=off  block_type=register
  Out1 : Outport
  wires:
  Register7/1 -> Out1/1
  In1/1 -> Register1/1
  Register5/1 -> Register7/1
  Register1/1 -> Register5/1

== system ar_lht_hw_target/AR_LHT_HW/DUT/Algorithm/AlgorithmDUT/Registers3 ==
  In1 : Inport
  Register1 : xbsIndex_r4/Register  init=0  rst=off  en=off  dbl_ovrd=off  block_type=register
  Register5 : xbsIndex_r4/Register  init=0  rst=off  en=off  dbl_ovrd=off  block_type=register
  Register7 : xbsIndex_r4/Register  init=0  rst=off  en=off  dbl_ovrd=off  block_type=register
  Out1 : Outport
  wires:
  Register5/1 -> Register7/1
  In1/1 -> Register1/1
  Register7/1 -> Out1/1
  Register1/1 -> Register5/1

== system ar_lht_hw_target/AR_LHT_HW/DUT/Algorithm/AlgorithmDUT/Registers4 ==
  In1 : Inport
  Register1 : xbsIndex_r4/Register  init=0  rst=off  en=off  dbl_ovrd=off  block_type=register
  Register5 : xbsIndex_r4/Register  init=0  rst=off  en=off  dbl_ovrd=off  block_type=register
  Register7 : xbsIndex_r4/Register  init=0  rst=off  en=off  dbl_ovrd=off  block_type=register
  Out1 : Outport
  wires:
  Register1/1 -> Register5/1
  Register5/1 -> Register7/1
  In1/1 -> Register1/1
  Register7/1 -> Out1/1

== system ar_lht_hw_target/AR_LHT_HW/DUT/Algorithm/AlgorithmDUT/Registers5 ==
  In1 : Inport
  Register1 : xbsIndex_r4/Register  init=0  rst=off  en=off  dbl_ovrd=off  block_type=register
  Register5 : xbsIndex_r4/Register  init=0  rst=off  en=off  dbl_ovrd=off  block_type=register
  Register7 : xbsIndex_r4/Register  init=0  rst=off  en=off  dbl_ovrd=off  block_type=register
  Out1 : Outport
  wires:
  Register7/1 -> Out1/1
  In1/1 -> Register1/1
  Register5/1 -> Register7/1
  Register1/1 -> Register5/1

== system ar_lht_hw_target/AR_LHT_HW/DUT/Algorithm/AlgorithmDUT/Registers6 ==
  In1 : Inport
  Register5 : xbsIndex_r4/Register  init=0  rst=off  en=off  dbl_ovrd=off  block_type=register
  Register7 : xbsIndex_r4/Register  init=0  rst=off  en=off  dbl_ovrd=off  block_type=register
  Out1 : Outport
  wires:
  Register7/1 -> Out1/1
  In1/1 -> Register5/1
  Register5/1 -> Register7/1

== system ar_lht_hw_target/AR_LHT_HW/DUT/Algorithm/AlgorithmDUT/Registers7 ==
  In1 : Inport
  Register{1..7} (7 alike) : xbsIndex_r4/Register  init=0  rst=off  en=off  dbl_ovrd=off  block_type=register
  Out1 : Outport
  wires:
  Register4/1 -> Register3/1
  Register3/1 -> Register2/1
  Register2/1 -> Register1/1
  Register7/1 -> Register6/1
  In1/1 -> Register4/1
  Register5/1 -> Register7/1
  Register1/1 -> Register5/1
  Register6/1 -> Out1/1

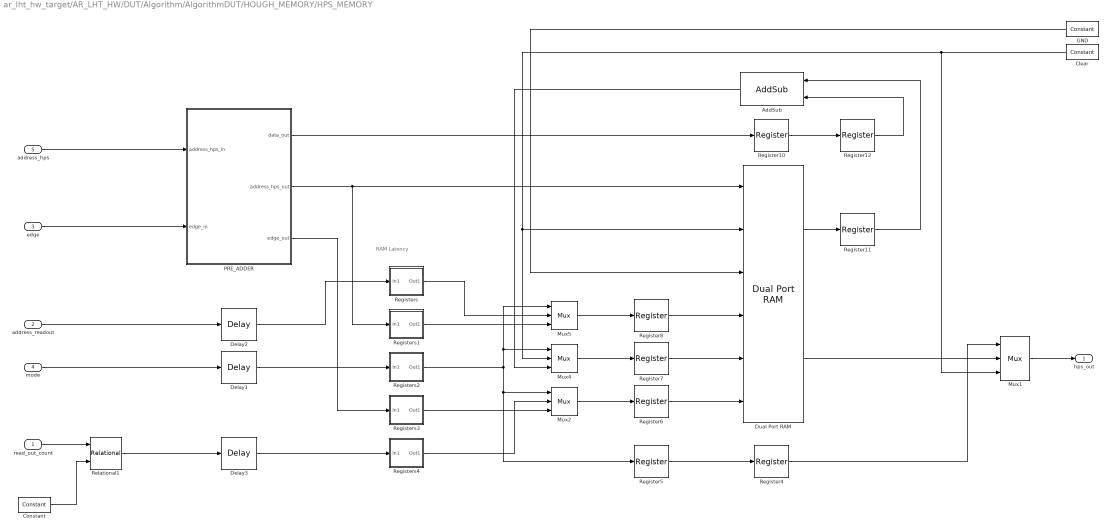
== system ar_lht_hw_target/AR_LHT_HW/DUT/Algorithm/AlgorithmDUT/HOUGH_MEMORY/HPS_MEMORY ==
  note: RAM Latency
  read_out_count : Inport
  address_readout : Inport  Port=2
  edge : Inport  Port=3
  mode : Inport  Port=4
  address_hps : Inport  Port=5
  AddSub : xbsIndex_r4/AddSub  mode=Addition  use_carryin=off  use_carryout=off  en=off  latency=1  precision=User Defined  arith_type=Unsigned  n_bits=ceil(log2(maxRho*2))  bin_pt=0  quantization=Truncate  overflow=Wrap  use_behavioral_HDL=off  hw_selection=Fabric  pipelined=off  dbl_ovrd=off  block_type=addsub
  Clear : xbsIndex_r4/Constant  const=0  gui_display_data_type=Fixed-point  arith_type=Unsigned  n_bits=18  bin_pt=0  preci_type=Single  exp_width=8  frac_width=24  explicit_period=on  period=T  equ=P=C  opselect=C  inp2=PCIN>>17  opr=+  inp1=P  carry=CIN  dbl_ovrd=off  block_type=constant
  Constant : xbsIndex_r4/Constant  const=R-1  gui_display_data_type=Fixed-point  arith_type=Unsigned  n_bits=ceil(log2(R))  bin_pt=0  preci_type=Single  exp_width=8  frac_width=24  explicit_period=on  period=T  equ=P=C  opselect=C  inp2=PCIN>>17  opr=+  inp1=P  carry=CIN  dbl_ovrd=off  block_type=constant
  Delay1 : xbsIndex_r4/Delay  rst=off  infoeditControl=Selection of Reset will increase slice count due to use of real FFs and instead of SRLs  en=off  latency=7  reg_retiming=off  dbl_ovrd=off  block_type=delay
  Delay2 : xbsIndex_r4/Delay  rst=off  infoeditControl=Selection of Reset will increase slice count due to use of real FFs and instead of SRLs  en=off  latency=7  reg_retiming=off  dbl_ovrd=off  block_type=delay
  Delay3 : xbsIndex_r4/Delay  rst=off  infoeditControl=Selection of Reset will increase slice count due to use of real FFs and instead of SRLs  en=off  latency=7  reg_retiming=off  dbl_ovrd=off  block_type=delay
  Dual Port RAM : xbsIndex_r4/Dual Port RAM  depth=K*maxRho*2  initVector=0  distributed_mem=Block RAM  init_a=0  init_b=0  rst_a=off  rst_b=off  en_a=off  en_b=off  latency=1  write_mode_A=Read Before Write  write_mode_B=Read Before Write  optimize=Area  dbl_ovrd=off  block_type=dpram
  GND : xbsIndex_r4/Constant  const=0  gui_display_data_type=Boolean  arith_type=Boolean  n_bits=18  bin_pt=0  preci_type=Single  exp_width=8  frac_width=24  explicit_period=on  period=T  equ=P=C  opselect=C  inp2=PCIN>>17  opr=+  inp1=P  carry=CIN  dbl_ovrd=off  block_type=constant
  Mux1 : xbsIndex_r4/Mux  inputs=2  en=off  latency=1  precision=Full  arith_type=Unsigned  n_bits=16  bin_pt=14  quantization=Truncate  overflow=Wrap  dbl_ovrd=off  block_type=mux
  Mux2 : xbsIndex_r4/Mux  inputs=2  en=off  latency=0  precision=Full  arith_type=Unsigned  n_bits=16  bin_pt=14  quantization=Truncate  overflow=Wrap  dbl_ovrd=off  block_type=mux
  Mux4 : xbsIndex_r4/Mux  inputs=2  en=off  latency=0  precision=Full  arith_type=Unsigned  n_bits=16  bin_pt=14  quantization=Truncate  overflow=Wrap  dbl_ovrd=off  block_type=mux
  Mux5 : xbsIndex_r4/Mux  inputs=2  en=off  latency=0  precision=Full  arith_type=Unsigned  n_bits=16  bin_pt=14  quantization=Truncate  overflow=Wrap  dbl_ovrd=off  block_type=mux
  PRE_ADDER : Subsystem
  Register{4..8,10..12} (8 alike) : xbsIndex_r4/Register  init=0  rst=off  en=off  dbl_ovrd=off  block_type=register
  Registers : Subsystem
  Registers1 : Subsystem
  Registers2 : Subsystem
  Registers3 : Subsystem
  Registers4 : Subsystem
  Relational1 : xbsIndex_r4/Relational  mode=a=b  op_type=Bool  en=off  latency=0  dbl_ovrd=off  block_type=relational
  hps_out : Outport
  wires:
  Register4/1 -> Mux1/1
  Constant/1 -> Relational1/2
  Mux1/1 -> hps_out/1
  Clear/1 -> Dual Port RAM/2, Mux4/2, Mux1/3
  Dual Port RAM/2 -> Mux1/2
  Register5/1 -> Register4/1
  Register6/1 -> Dual Port RAM/6
  Register7/1 -> Dual Port RAM/5
  Mux2/1 -> Register6/1
  Mux4/1 -> Register7/1
  Mux5/1 -> Register8/1
  Register8/1 -> Dual Port RAM/4
  GND/1 -> Dual Port RAM/3
  read_out_count/1 -> Relational1/1
  address_hps/1 -> PRE_ADDER/1(address_hps_in)
  edge/1 -> PRE_ADDER/2(edge_in)
  PRE_ADDER/2(address_hps_out) -> Registers1/1(In1), Dual Port RAM/1
  PRE_ADDER/3(edge_out) -> Registers3/1(In1)
  Dual Port RAM/1 -> Register11/1
  PRE_ADDER/1(data_out) -> Register10/1
  AddSub/1 -> Mux4/3
  mode/1 -> Delay1/1
  Relational1/1 -> Delay3/1
  address_readout/1 -> Delay2/1
  Registers4/1(Out1) -> Mux2/2
  Registers3/1(Out1) -> Mux2/3
  Registers2/1(Out1) -> Register5/1, Mux2/1, Mux5/1, Mux4/1
  Registers/1(Out1) -> Mux5/2
  Registers1/1(Out1) -> Mux5/3
  Register10/1 -> Register12/1
  Delay2/1 -> Registers/1(In1)
  Delay1/1 -> Registers2/1(In1)
  Delay3/1 -> Registers4/1(In1)
  Register11/1 -> AddSub/1
  Register12/1 -> AddSub/2

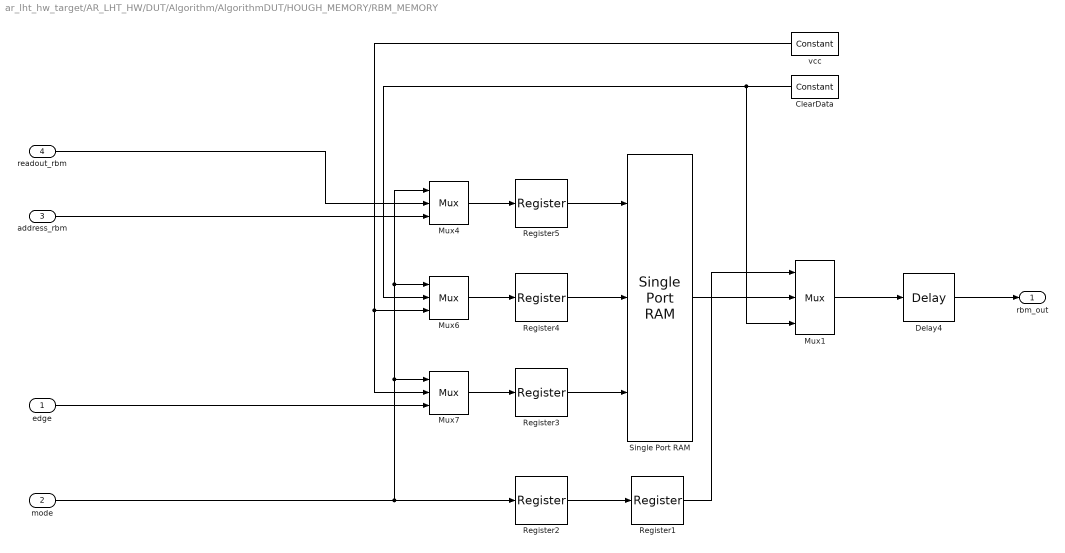
== system ar_lht_hw_target/AR_LHT_HW/DUT/Algorithm/AlgorithmDUT/HOUGH_MEMORY/RBM_MEMORY ==
  edge : Inport
  mode : Inport  Port=2
  address_rbm : Inport  Port=3
  readout_rbm : Inport  Port=4
  ClearData : xbsIndex_r4/Constant  const=0  gui_display_data_type=Boolean  arith_type=Boolean  n_bits=9  bin_pt=0  preci_type=Single  exp_width=8  frac_width=24  explicit_period=on  period=T  equ=P=C  opselect=C  inp2=PCIN>>17  opr=+  inp1=P  carry=CIN  dbl_ovrd=off  block_type=constant
  Delay4 : xbsIndex_r4/Delay  rst=off  infoeditControl=Selection of Reset will increase slice count due to use of real FFs and instead of SRLs  en=off  latency=10  reg_retiming=off  dbl_ovrd=off  block_type=delay
  Mux1 : xbsIndex_r4/Mux  inputs=2  en=off  latency=1  precision=User Defined  arith_type=Unsigned  n_bits=1  bin_pt=0  quantization=Truncate  overflow=Wrap  dbl_ovrd=off  block_type=mux
  Mux4 : xbsIndex_r4/Mux  inputs=2  en=off  latency=0  precision=Full  arith_type=Unsigned  n_bits=16  bin_pt=14  quantization=Truncate  overflow=Wrap  dbl_ovrd=off  block_type=mux
  Mux6 : xbsIndex_r4/Mux  inputs=2  en=off  latency=0  precision=Full  arith_type=Unsigned  n_bits=16  bin_pt=14  quantization=Truncate  overflow=Wrap  dbl_ovrd=off  block_type=mux
  Mux7 : xbsIndex_r4/Mux  inputs=2  en=off  latency=0  precision=Full  arith_type=Unsigned  n_bits=16  bin_pt=14  quantization=Truncate  overflow=Wrap  dbl_ovrd=off  block_type=mux
  Register{1..5} (5 alike) : xbsIndex_r4/Register  init=0  rst=off  en=off  dbl_ovrd=off  block_type=register
  Single Port RAM : xbsIndex_r4/Single Port RAM  depth=(maxTheta+deltaTheta)*maxRho*2  initVector=0  distributed_mem=Block RAM  write_mode=Read Before Write  rst=off  init_reg=0  en=off  latency=1  optimize=Area  dbl_ovrd=off  block_type=spram
  vcc : xbsIndex_r4/Constant  const=1  gui_display_data_type=Boolean  arith_type=Boolean  n_bits=9  bin_pt=0  preci_type=Single  exp_width=8  frac_width=24  explicit_period=on  period=T  equ=P=C  opselect=C  inp2=PCIN>>17  opr=+  inp1=P  carry=CIN  dbl_ovrd=off  block_type=constant
  rbm_out : Outport
  wires:
  readout_rbm/1 -> Mux4/2
  address_rbm/1 -> Mux4/3
  Mux4/1 -> Register5/1
  Mux7/1 -> Register3/1
  Mux6/1 -> Register4/1
  ClearData/1 -> Mux6/2, Mux1/3
  edge/1 -> Mux7/3
  vcc/1 -> Mux6/3, Mux7/2
  Mux1/1 -> Delay4/1
  Single Port RAM/1 -> Mux1/2
  mode/1 -> Register2/1, Mux4/1, Mux6/1, Mux7/1
  Register1/1 -> Mux1/1
  Register2/1 -> Register1/1
  Register3/1 -> Single Port RAM/3
  Register4/1 -> Single Port RAM/2
  Register5/1 -> Single Port RAM/1
  Delay4/1 -> rbm_out/1
